simulink model "PID_VELOCIDAD_MOTORDC_ANTI_WINDUP_2022"  (R2022b)
settings: Solver=ode1  StartTime=0.0  StopTime=inf  FixedStep=0.01  RelTol=1e-3
undefined symbols (not defined in the file): G1, kd, ki, kp
libraries: arduinolib x3, fod x2, arduinosensorlib x1, simulink x1
settings Model: ExtModeTrigDuration=2  Creator=Mario  LastModifiedBy=Mario
settings OptimizationCC: EnhancedBackFolding=on  PassReuseOutputArgsThreshold=0  MaxStackSize=64  OptimizeBlockOrder=speed  DifferentSizesBufferReuse=on  OptimizationCustomize=off
settings DebuggingCC: ParameterTunabilityLossMsg=error
settings HardwareCC: ProdBitPerPointer=32  ProdBitPerSizeT=32  ProdBitPerPtrDiffT=32  ProdLargestAtomicInteger=Long  ProdLargestAtomicFloat=Double  ProdWordSize=32  ProdHWDeviceType=ARM Compatible->ARM Cortex  UseEmbeddedCoderFeatures=off
settings SFSimCC: MATLABDynamicMemAlloc=off
settings RTWCC: Description=Embedded Coder  SystemTargetFile=ert.tlc  HardwareBoard=Arduino Due  TLCOptions=-aInlineSetEventsForThisBaseRateFcn=TLC_FALSE -aSuppressMultiTaskScheduler=TLC_FALSE -aRateBasedStepFcn=1  TemplateMakefile=ert_default_tmf  Toolchain=Arduino ARM  BuildConfiguration=Faster Runs
settings CodeAppCC: ForceParamTrailComments=on  OperatorAnnotations=on
settings ERTTargetCC: ERTCustomFileBanners=off  SupportContinuousTime=on  SupportNonInlinedSFcns=on  RemoveResetFunc=off  SupportVariableSizeSignals=on  ModelStepFunctionPrototypeControlCompliant=off  ExtModeTransport=3  ExtModeStaticAlloc=on  ExtModeAutomaticAllocSize=off  ExtModeStaticAllocSize=24576  ExtModeMexFile=ext_xcp  ExtModeIntrfLevel=Level2 - Open

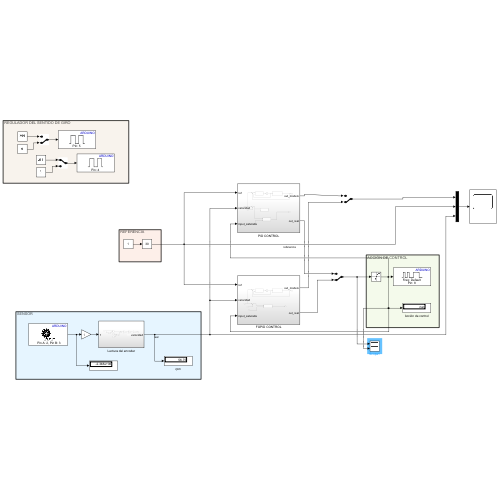
[thumbnail: Simulink's stored preview of the top-level diagram]
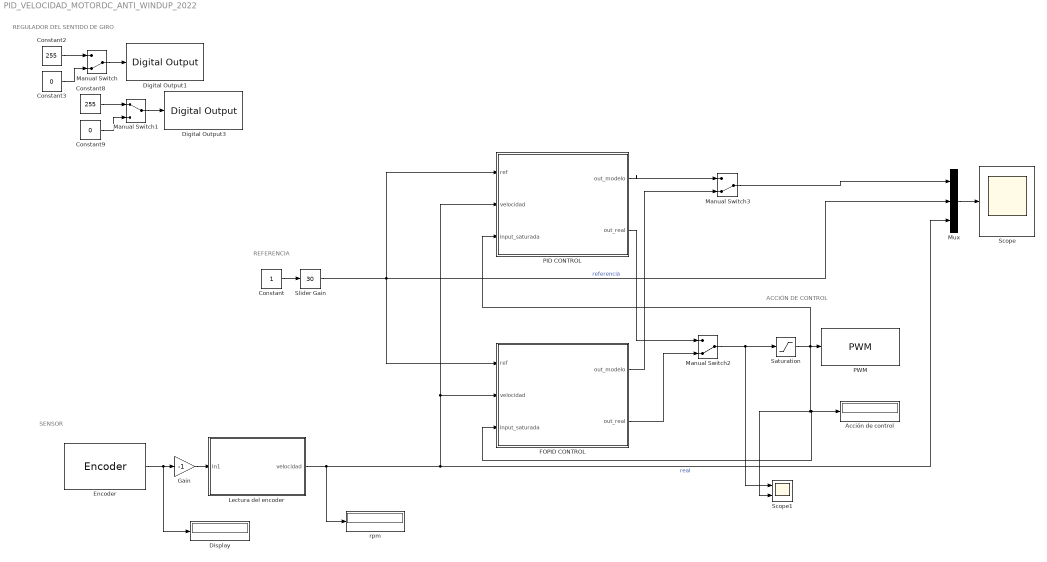
== system PID_VELOCIDAD_MOTORDC_ANTI_WINDUP_2022 ==
  note: SENSOR
  note: REFERENCIA
  note: REGULADOR DEL SENTIDO DE GIRO
  note: ACCIÓN DE CONTROL
  Acción de control : Display
  Constant : Constant
  Constant2 : Constant  Value=255
  Constant3 : Constant  Value=0
  Constant8 : Constant  Value=255
  Constant9 : Constant  Value=0
  Digital Output1 : arduinolib/Digital Output  pinNumber=5  Direction=output  blockPlatform=arduino
  Digital Output3 : arduinolib/Digital Output  pinNumber=4  Direction=output  blockPlatform=arduino
  Display : Display
  Encoder : arduinosensorlib/Encoder  InputA=2  InputB=3  Mode=No reset  SampleTime=-1
  FOPID CONTROL : Subsystem
  Gain : Gain  Gain=-1
  Lectura del encoder : Subsystem
  Manual Switch : ManualSwitch  CurrentSetting=0
  Manual Switch1 : ManualSwitch
  Manual Switch2 : ManualSwitch  CurrentSetting=0
  Manual Switch3 : ManualSwitch  CurrentSetting=0
  Mux : Mux  Inputs=3
  PID CONTROL : Subsystem
  PWM : arduinolib/PWM  pinNumber=8  frequencyType=Default  desiredFrequency=490.2  achievableFrequency=490.2
  Saturation : Saturate  UpperLimit=255  LowerLimit=0
  Scope : Scope
  Scope1 : Scope  NumInputPorts=2
  Slider Gain : simulink/Math Operations/Slider Gain  gain=30  low=0  high=70
  rpm : Display
  wires:
  Constant3/1 -> Manual Switch/2
  Constant8/1 -> Manual Switch1/1
  Constant9/1 -> Manual Switch1/2
  Constant2/1 -> Manual Switch/1
  Manual Switch/1 -> Digital Output1/1
  Manual Switch1/1 -> Digital Output3/1
  Lectura del encoder/1(velocidad) -> Mux/3, FOPID CONTROL/2(velocidad), PID CONTROL/2(velocidad), rpm/1  "real"
  Encoder/1 -> Display/1, Gain/1
  Slider Gain/1 -> FOPID CONTROL/1(ref), PID CONTROL/1(ref), Mux/2  "referencia"
  Mux/1 -> Scope/1
  Constant/1 -> Slider Gain/1
  Saturation/1 -> PID CONTROL/3(input_saturada), FOPID CONTROL/3(input_saturada), Acción de control/1, Scope1/2, PWM/1
  PID CONTROL/2(out_real) -> Manual Switch2/1
  FOPID CONTROL/2(out_real) -> Manual Switch2/2
  PID CONTROL/1(out_modelo) -> Manual Switch3/1
  FOPID CONTROL/1(out_modelo) -> Manual Switch3/2
  Manual Switch3/1 -> Mux/1
  Gain/1 -> Lectura del encoder/1(In1)
  Manual Switch2/1 -> Scope1/1, Saturation/1

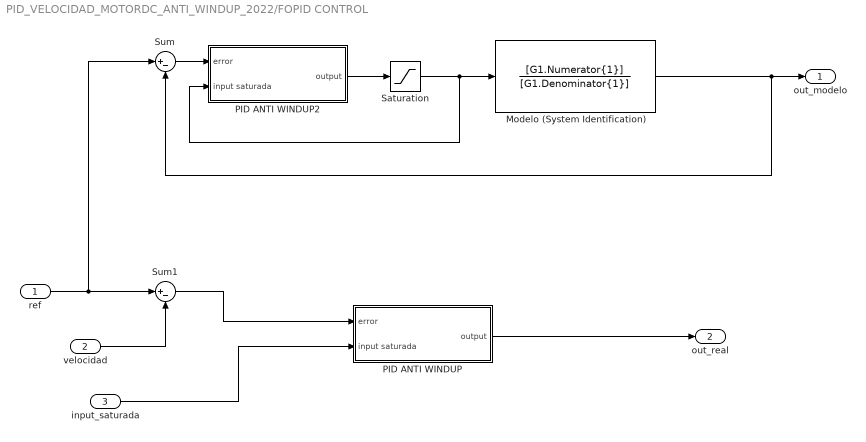
== system PID_VELOCIDAD_MOTORDC_ANTI_WINDUP_2022/FOPID CONTROL ==
  ref : Inport
  velocidad : Inport  Port=2
  input_saturada : Inport  Port=3
  Modelo (System Identification) : TransferFcn  Numerator=[G1.Numerator{1}]  Denominator=[G1.Denominator{1}]
  PID ANTI WINDUP : Subsystem
  PID ANTI WINDUP2 : Subsystem
  Saturation : Saturate
  Sum : Sum  Inputs=|+-
  Sum1 : Sum  Inputs=|+-
  out_modelo : Outport
  out_real : Outport  Port=2
  wires:
  Modelo (System Identification)/1 -> out_modelo/1, Sum/2
  ref/1 -> Sum/1, Sum1/1
  velocidad/1 -> Sum1/2
  Sum1/1 -> PID ANTI WINDUP/1(error)
  PID ANTI WINDUP2/1(output) -> Saturation/1
  Sum/1 -> PID ANTI WINDUP2/1(error)
  input_saturada/1 -> PID ANTI WINDUP/2(input saturada)
  PID ANTI WINDUP/1(output) -> out_real/1
  Saturation/1 -> Modelo (System Identification)/1, PID ANTI WINDUP2/2(input saturada)

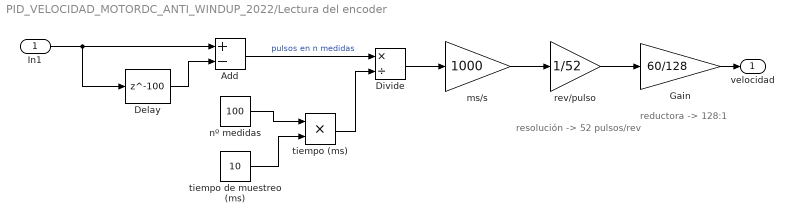
== system PID_VELOCIDAD_MOTORDC_ANTI_WINDUP_2022/Lectura del encoder ==
  note: reductora -> 128:1
  note: resolución -> 52 pulsos/rev
  In1 : Inport
  Add : Sum  Inputs=+-
  Delay : Delay  DelayLength=100
  Divide : Product  Inputs=*/
  Gain : Gain  Gain=60/128
  ms/s : Gain  Gain=1000
  nº medidas : Constant  Value=100
  rev/pulso : Gain  Gain=1/52
  tiempo (ms) : Product  Inputs=**
  tiempo de muestreo (ms) : Constant  Value=10
  velocidad : Outport
  wires:
  Delay/1 -> Add/2
  Divide/1 -> ms/s/1
  In1/1 -> Delay/1, Add/1
  nº medidas/1 -> tiempo (ms)/1
  Add/1 -> Divide/1  "pulsos en n medidas"
  rev/pulso/1 -> Gain/1
  Gain/1 -> velocidad/1
  ms/s/1 -> rev/pulso/1
  tiempo de muestreo (ms)/1 -> tiempo (ms)/2
  tiempo (ms)/1 -> Divide/2

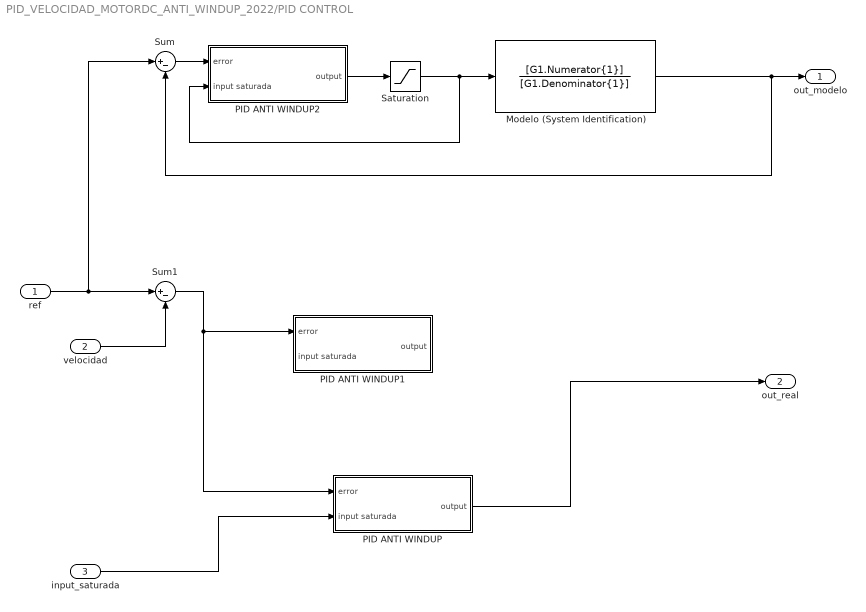
== system PID_VELOCIDAD_MOTORDC_ANTI_WINDUP_2022/PID CONTROL ==
  ref : Inport
  velocidad : Inport  Port=2
  input_saturada : Inport  Port=3
  Modelo (System Identification) : TransferFcn  Numerator=[G1.Numerator{1}]  Denominator=[G1.Denominator{1}]
  PID ANTI WINDUP : Subsystem
  PID ANTI WINDUP1 : Subsystem
  PID ANTI WINDUP2 : Subsystem
  Saturation : Saturate
  Sum : Sum  Inputs=|+-
  Sum1 : Sum  Inputs=|+-
  out_modelo : Outport
  out_real : Outport  Port=2
  wires:
  Modelo (System Identification)/1 -> out_modelo/1, Sum/2
  ref/1 -> Sum/1, Sum1/1
  velocidad/1 -> Sum1/2
  Sum1/1 -> PID ANTI WINDUP/1(error), PID ANTI WINDUP1/1(error)
  PID ANTI WINDUP2/1(output) -> Saturation/1
  Sum/1 -> PID ANTI WINDUP2/1(error)
  input_saturada/1 -> PID ANTI WINDUP/2(input saturada)
  PID ANTI WINDUP/1(output) -> out_real/1
  Saturation/1 -> Modelo (System Identification)/1, PID ANTI WINDUP2/2(input saturada)

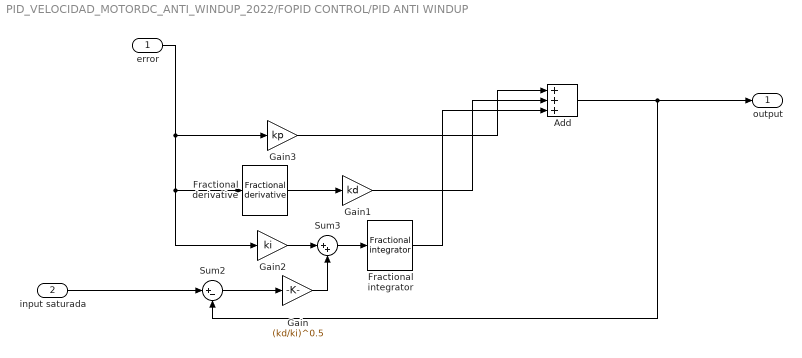
== system PID_VELOCIDAD_MOTORDC_ANTI_WINDUP_2022/FOPID CONTROL/PID ANTI WINDUP ==
  error : Inport
  input saturada : Inport  Port=2
  Add : Sum  Inputs=+++
  Fractional derivative : fod/Fractional derivative  gam=0.85  ww=[0.001; 500]  n=5  nFod=off
      settings: SourceProductName=FOMCON Toolbox
  Fractional integrator : fod/Fractional integrator  gam=0.95  ww=[0.001; 500]  n=5  nFod=off
      settings: SourceProductName=FOMCON Toolbox
  Gain : Gain  Gain=(kd/ki)^0.5
  Gain1 : Gain  Gain=kd
  Gain2 : Gain  Gain=ki
  Gain3 : Gain  Gain=kp
  Sum2 : Sum  Inputs=|+-
  Sum3 : Sum  Inputs=|++
  output : Outport
  wires:
  Gain2/1 -> Sum3/1
  Add/1 -> output/1, Sum2/2
  error/1 -> Fractional derivative/1, Gain2/1, Gain3/1
  Gain1/1 -> Add/2
  Gain3/1 -> Add/1
  Fractional derivative/1 -> Gain1/1
  Sum2/1 -> Gain/1
  Sum3/1 -> Fractional integrator/1
  Gain/1 -> Sum3/2
  input saturada/1 -> Sum2/1
  Fractional integrator/1 -> Add/3

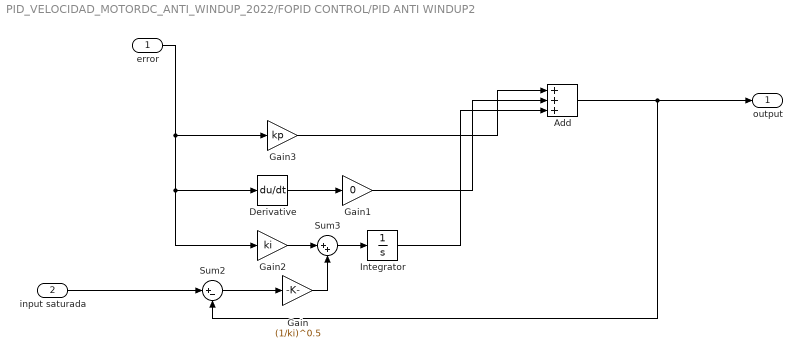
== system PID_VELOCIDAD_MOTORDC_ANTI_WINDUP_2022/FOPID CONTROL/PID ANTI WINDUP2 ==
  error : Inport
  input saturada : Inport  Port=2
  Add : Sum  Inputs=+++
  Derivative : Derivative
  Gain : Gain  Gain=(1/ki)^0.5
  Gain1 : Gain  Gain=0
  Gain2 : Gain  Gain=ki
  Gain3 : Gain  Gain=kp
  Integrator : Integrator
  Sum2 : Sum  Inputs=|+-
  Sum3 : Sum  Inputs=|++
  output : Outport
  wires:
  Gain2/1 -> Sum3/1
  Add/1 -> output/1, Sum2/2
  error/1 -> Gain2/1, Derivative/1, Gain3/1
  Gain1/1 -> Add/2
  Gain3/1 -> Add/1
  Derivative/1 -> Gain1/1
  Sum2/1 -> Gain/1
  Integrator/1 -> Add/3
  Sum3/1 -> Integrator/1
  Gain/1 -> Sum3/2
  input saturada/1 -> Sum2/1

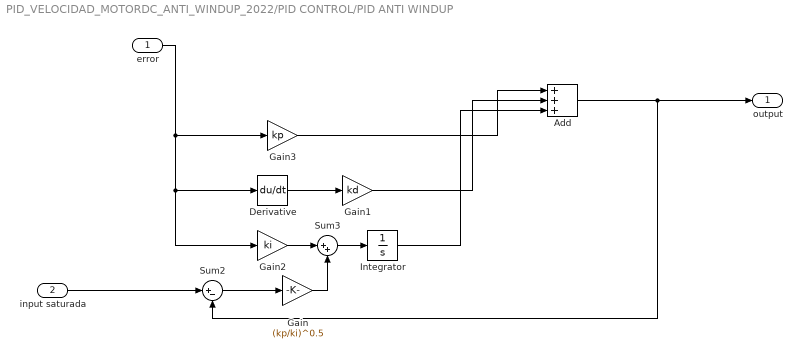
== system PID_VELOCIDAD_MOTORDC_ANTI_WINDUP_2022/PID CONTROL/PID ANTI WINDUP ==
  error : Inport
  input saturada : Inport  Port=2
  Add : Sum  Inputs=+++
  Derivative : Derivative
  Gain : Gain  Gain=(kp/ki)^0.5
  Gain1 : Gain  Gain=kd
  Gain2 : Gain  Gain=ki
  Gain3 : Gain  Gain=kp
  Integrator : Integrator
  Sum2 : Sum  Inputs=|+-
  Sum3 : Sum  Inputs=|++
  output : Outport
  wires:
  Gain2/1 -> Sum3/1
  Add/1 -> output/1, Sum2/2
  error/1 -> Gain2/1, Derivative/1, Gain3/1
  Gain1/1 -> Add/2
  Gain3/1 -> Add/1
  Derivative/1 -> Gain1/1
  Sum2/1 -> Gain/1
  Integrator/1 -> Add/3
  Sum3/1 -> Integrator/1
  Gain/1 -> Sum3/2
  input saturada/1 -> Sum2/1

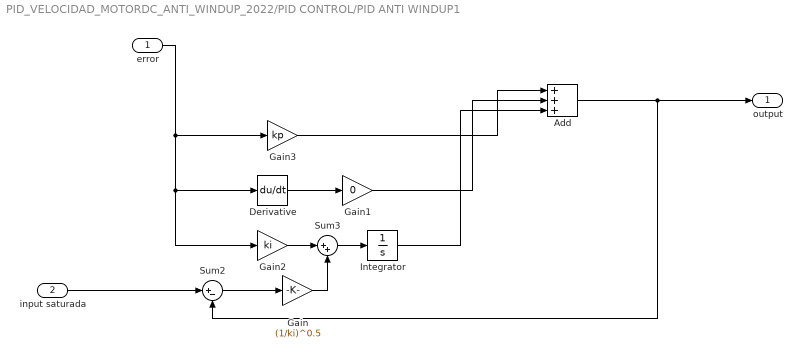
== system PID_VELOCIDAD_MOTORDC_ANTI_WINDUP_2022/PID CONTROL/PID ANTI WINDUP1 ==
  error : Inport
  input saturada : Inport  Port=2
  Add : Sum  Inputs=+++
  Derivative : Derivative
  Gain : Gain  Gain=(1/ki)^0.5
  Gain1 : Gain  Gain=0
  Gain2 : Gain  Gain=ki
  Gain3 : Gain  Gain=kp
  Integrator : Integrator
  Sum2 : Sum  Inputs=|+-
  Sum3 : Sum  Inputs=|++
  output : Outport
  wires:
  Gain2/1 -> Sum3/1
  Add/1 -> output/1, Sum2/2
  error/1 -> Gain2/1, Derivative/1, Gain3/1
  Gain1/1 -> Add/2
  Gain3/1 -> Add/1
  Derivative/1 -> Gain1/1
  Sum2/1 -> Gain/1
  Integrator/1 -> Add/3
  Sum3/1 -> Integrator/1
  Gain/1 -> Sum3/2
  input saturada/1 -> Sum2/1

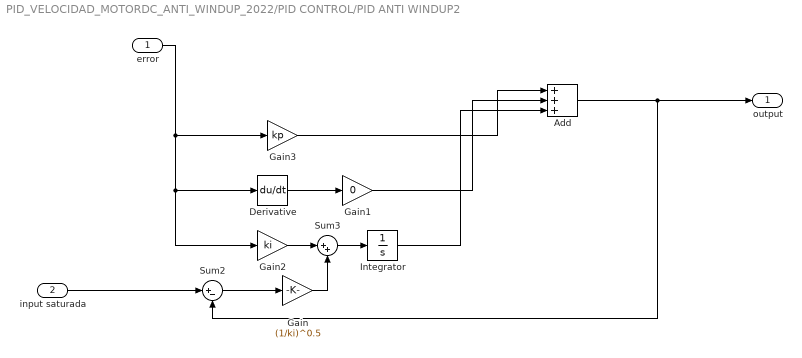
== system PID_VELOCIDAD_MOTORDC_ANTI_WINDUP_2022/PID CONTROL/PID ANTI WINDUP2 ==
  error : Inport
  input saturada : Inport  Port=2
  Add : Sum  Inputs=+++
  Derivative : Derivative
  Gain : Gain  Gain=(1/ki)^0.5
  Gain1 : Gain  Gain=0
  Gain2 : Gain  Gain=ki
  Gain3 : Gain  Gain=kp
  Integrator : Integrator
  Sum2 : Sum  Inputs=|+-
  Sum3 : Sum  Inputs=|++
  output : Outport
  wires:
  Gain2/1 -> Sum3/1
  Add/1 -> output/1, Sum2/2
  error/1 -> Gain2/1, Derivative/1, Gain3/1
  Gain1/1 -> Add/2
  Gain3/1 -> Add/1
  Derivative/1 -> Gain1/1
  Sum2/1 -> Gain/1
  Integrator/1 -> Add/3
  Sum3/1 -> Integrator/1
  Gain/1 -> Sum3/2
  input saturada/1 -> Sum2/1
